simulink library "cylinderVolume_ul"  (R2018b)
settings: Solver=VariableStepAuto  StartTime=0.0  StopTime=10.0  RelTol=1e-3
settings Model: Creator=asiddiq2  LastModifiedBy=Ayaz

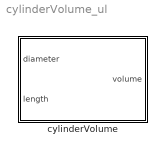
== system cylinderVolume_ul ==
  cylinderVolume : Subsystem

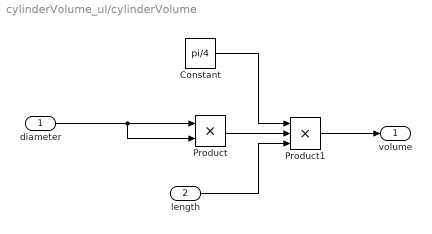
== system cylinderVolume_ul/cylinderVolume ==
  diameter : Inport
  length : Inport  Port=2
  Constant : Constant  Value=pi/4
  Product : Product
  Product1 : Product  Inputs=3
  volume : Outport
  wires:
  diameter/1 -> Product/2, Product/1
  Constant/1 -> Product1/1
  Product/1 -> Product1/2
  length/1 -> Product1/3
  Product1/1 -> volume/1
